simulink model "notch_tb_varTs"  (R2021a)
settings: Solver=VariableStepAuto  StartTime=0.0  StopTime=0.01  RelTol=1e-3
values from neighbouring files (symbols this model uses):
  FPGA_CLK_MHZ = 125    [lowpass_modelcomp_v1_0_setup.m]    (also in notch_modelcomp_v1_0_setup.m)
  maxSampleRate = 1e6    (= 1000000)    [lowpass_modelcomp_v1_0_setup.m]    (also in notch_modelcomp_v1_0_setup.m)
  notch_A0 = al0/be0    (= 0.984901734501)    [notch_modelcomp_v1_0_setup.m]
  notch_A1 = al1/be0    (= -1.87493826905)    [notch_modelcomp_v1_0_setup.m]
  notch_A2 = al2/be0    (= 0.984901734501)    [notch_modelcomp_v1_0_setup.m]
  notch_B1 = be1/be0    (= -1.87493826905)    [notch_modelcomp_v1_0_setup.m]
  notch_B2 = be2/be0    (= 0.969803469002)    [notch_modelcomp_v1_0_setup.m]
  samplePeriod = 1./SampleRate    (= 1e-05)    [lowpass_modelcomp_v1_0_setup.m]    (also in notch_modelcomp_v1_0_setup.m)
undefined symbols (not defined in the file or in its folder): xc7z030sbg485
libraries: hdlBasic x36, simulink x1, vmcUtilities x1, hdlUtilities x1
settings Model: Creator=osboxes  LastModifiedBy=valbas
settings SolverCC: AlgebraicLoopSolver=TrustRegion
settings DebuggingCC: SFMachineParentedDataDiag=warning

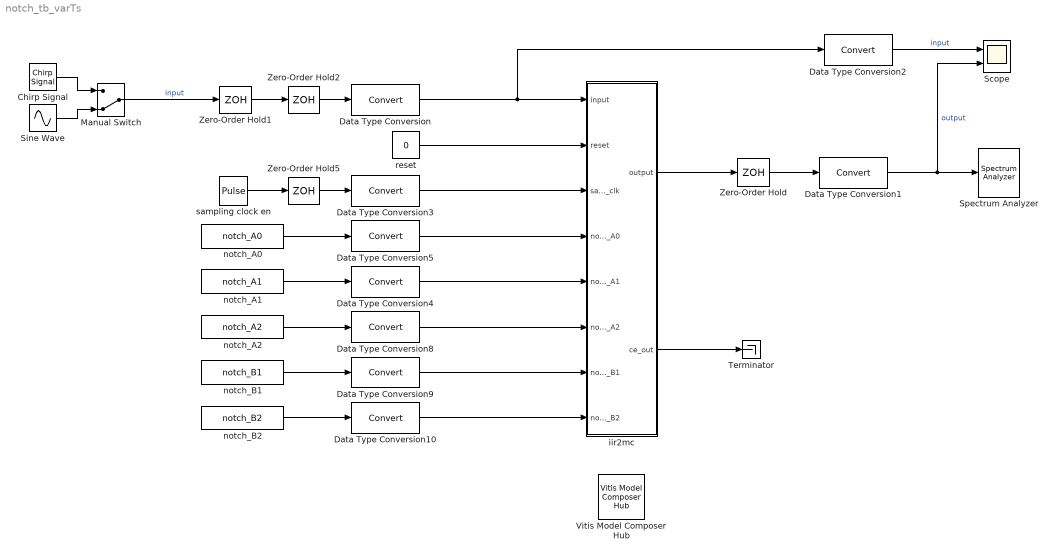
== system notch_tb_varTs ==
  Chirp Signal : simulink/Sources/Chirp Signal  f1=1  T=5  f2=1000
  Data Type Conversion{,1..2,4..5,8..10} (8 alike) : DataTypeConversion  RndMeth=Round
  Data Type Conversion3 : DataTypeConversion
  Manual Switch : ManualSwitch  CurrentSetting=0
  Scope : Scope  NumInputPorts=2
  Sine Wave : Sin  Amplitude=0.5  Frequency=4950*2*pi  SampleTime=0
  Spectrum Analyzer : SpectrumAnalyzer
  Terminator : Terminator
  Vitis Model Composer Hub : vmcUtilities/Vitis Model Composer Hub  Tag=genX  CodeGeneration=off  SubsystemName=iir2mc  TargetDirectory=./code  ExportType=HDL  IpVendor=xilinx.com  IpLibrary=hls  IpVersion=1.0  IpHWLanguage=Verilog  AieCompilerOptions={}  AieSimulatorOptions={}  CreateTestbench=off  TestbenchStackSize=10  RunRtlSim=off  RunCSim=off  RunAieSim=off  AieSimTimeout=50000  RunAieSimProfiling=off  LaunchVitisAnalyzer=off  PlotOutput=off  RunX86Sim=off  X86SimTimeout=10  GenHwImage=off  GenLibadfXo=off  PlatformType=Not Specified  HwSystemType=Baremetal  HwValidationTarget=hw  ProjDevice=xc7z030sbg485-1  ProjDevicePart=xc7z030sbg485-1  SamplePeriod=-1  ClockFrequency=200  DataPathParallelism=1  xilinxfamily=zynq  part=xc7z030  speed=-1  package=sbg485  directory=./netlist/ip/iir2mc/src  testbench=off  incr_netlist=off  synthesis_tool=Vivado  clock_wrapper=Clock Enables  dbl_ovrd=According to Block Masks  dcm_input_clock_period=10  sysclk_period=1.e3/FPGA_CLK_MHZ  simulink_period=1/(FPGA_CLK_MHZ*1.e6)  eval_field=0  IPInfoJsonString="{\"HDLSubsystem\":{\"SubsystemName\":\"iir2mc\",\"IPName\":\"iir2mc\",\"IPLibrary\":\"Panda_ModelComp\",\"IPVendor\":\"MaxIV\",\"IPVersion\":\"1.0\",\"TargetDirectory\":\"./netlist\",\"SubsystemDir\":\"./netlist/ip/iir2mc\"}}"  LogFileName=''  NThreads=4
  Zero-Order Hold : ZeroOrderHold  SampleTime=1/(FPGA_CLK_MHZ*1.e6)
  Zero-Order Hold1 : ZeroOrderHold  SampleTime=samplePeriod
  Zero-Order Hold2 : ZeroOrderHold  SampleTime=1/(FPGA_CLK_MHZ*1.e6)
  Zero-Order Hold5 : ZeroOrderHold  SampleTime=1/(FPGA_CLK_MHZ*1.e6)
  iir2mc : Subsystem
  notch_A0 : Constant  Value=notch_A0  OutDataTypeStr=double  SampleTime=1/(FPGA_CLK_MHZ*1.e6)
  notch_A1 : Constant  Value=notch_A1  OutDataTypeStr=double  SampleTime=1/(FPGA_CLK_MHZ*1.e6)
  notch_A2 : Constant  Value=notch_A2  OutDataTypeStr=double  SampleTime=1/(FPGA_CLK_MHZ*1.e6)
  notch_B1 : Constant  Value=notch_B1  OutDataTypeStr=double  SampleTime=1/(FPGA_CLK_MHZ*1.e6)
  notch_B2 : Constant  Value=notch_B2  OutDataTypeStr=double  SampleTime=1/(FPGA_CLK_MHZ*1.e6)
  reset : Constant  Value=0  OutDataTypeStr=boolean  SampleTime=1/(FPGA_CLK_MHZ*1.e6)
  sampling clock en : DiscretePulseGenerator  PulseType=Time based  Period=samplePeriod  PulseWidth=100/(samplePeriod*maxSampleRate)
  wires:
  Zero-Order Hold/1 -> Data Type Conversion1/1
  Zero-Order Hold2/1 -> Data Type Conversion/1
  reset/1 -> iir2mc/2(reset)
  iir2mc/1(output) -> Zero-Order Hold/1
  iir2mc/2(ce_out) -> Terminator/1
  Zero-Order Hold5/1 -> Data Type Conversion3/1
  Data Type Conversion3/1 -> iir2mc/3(sample_clk)
  notch_A0/1 -> Data Type Conversion5/1
  Data Type Conversion5/1 -> iir2mc/4(notch_A0)
  notch_A1/1 -> Data Type Conversion4/1
  Data Type Conversion4/1 -> iir2mc/5(notch_A1)
  notch_A2/1 -> Data Type Conversion8/1
  Data Type Conversion8/1 -> iir2mc/6(notch_A2)
  notch_B1/1 -> Data Type Conversion9/1
  Data Type Conversion9/1 -> iir2mc/7(notch_B1)
  notch_B2/1 -> Data Type Conversion10/1
  Data Type Conversion10/1 -> iir2mc/8(notch_B2)
  sampling clock en/1 -> Zero-Order Hold5/1
  Data Type Conversion/1 -> Data Type Conversion2/1, iir2mc/1(input)
  Data Type Conversion1/1 -> Scope/2, Spectrum Analyzer/1  "output"
  Sine Wave/1 -> Manual Switch/2
  Chirp Signal/1 -> Manual Switch/1
  Data Type Conversion2/1 -> Scope/1  "input"
  Zero-Order Hold1/1 -> Zero-Order Hold2/1
  Manual Switch/1 -> Zero-Order Hold1/1  "input"

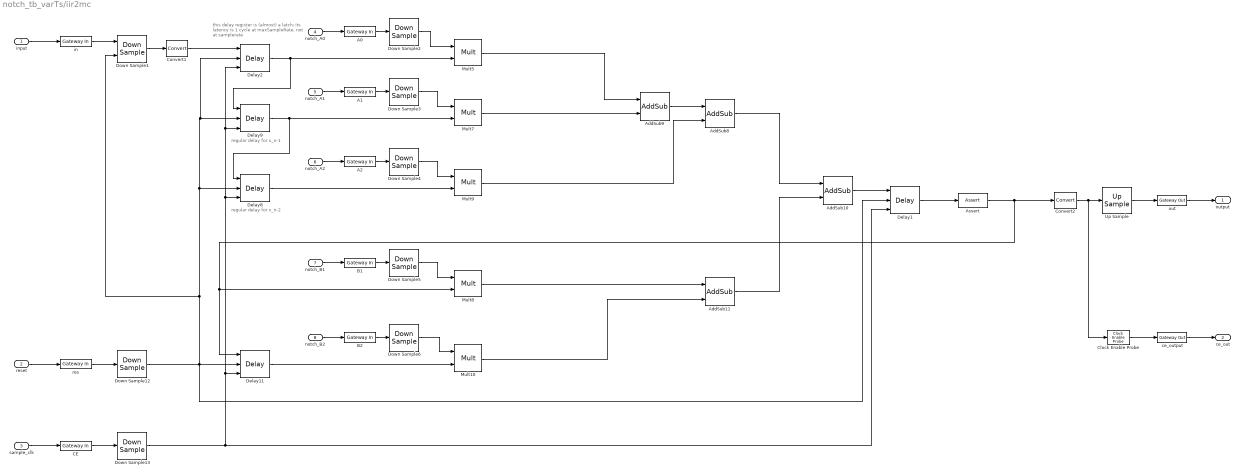
== system notch_tb_varTs/iir2mc ==
  note: regular delay for x_n-1
  note: this delay register is (almost) a latch;
      | its latency is 1 cycle at maxSampleRate,
      | not at samplerate
  note: regular delay for x_n-2
  input : Inport  OutDataTypeStr=fixdt(1,32,31)
  reset : Inport  Port=2
  sample_clk : Inport  Port=3  OutDataTypeStr=boolean
  notch_A0 : Inport  Port=4  OutDataTypeStr=single
  notch_A1 : Inport  Port=5  OutDataTypeStr=single
  notch_A2 : Inport  Port=6  OutDataTypeStr=single
  notch_B1 : Inport  Port=7  OutDataTypeStr=single
  notch_B2 : Inport  Port=8  OutDataTypeStr=single
  A0 : hdlBasic/Gateway In  gui_display_data_type=Floating-point  arith_type=Floating-point  n_bits=32  bin_pt=16  preci_type=Single  exp_width=8  frac_width=24  rows=1  columns=1  quantization="Round  (unbiased: +/- Inf)"  overflow=Saturate  period=1/(FPGA_CLK_MHZ*1.e6)  UseAsADC=off  ADCChannel='1'  interface=None  automatic_assignment=on  address_offset=hex2dec('00')  intf_name=''  intf_description=''  default_value=0  timing_constraint=None  locs_specified=off  LOCs={}  io_standard={}  inherit_from_input=off  hdl_port=on  XmcBlockStatus=1  maskContainerNames=group4  block_type=gatewayin  block_config=sysgen:gateway_in_config  block_width_w=590  block_height_w=620  block_width=640  block_height=850
  A1 : hdlBasic/Gateway In  gui_display_data_type=Floating-point  arith_type=Floating-point  n_bits=32  bin_pt=16  preci_type=Single  exp_width=8  frac_width=24  rows=1  columns=1  quantization="Round  (unbiased: +/- Inf)"  overflow=Saturate  period=1/(FPGA_CLK_MHZ*1.e6)  UseAsADC=off  ADCChannel='1'  interface=None  automatic_assignment=on  address_offset=hex2dec('00')  intf_name=''  intf_description=''  default_value=0  timing_constraint=None  locs_specified=off  LOCs={}  io_standard={}  inherit_from_input=off  hdl_port=on  XmcBlockStatus=1  maskContainerNames=group4  block_type=gatewayin  block_config=sysgen:gateway_in_config  block_width_w=590  block_height_w=620  block_width=640  block_height=850
  A2 : hdlBasic/Gateway In  gui_display_data_type=Floating-point  arith_type=Floating-point  n_bits=32  bin_pt=16  preci_type=Single  exp_width=8  frac_width=24  rows=1  columns=1  quantization="Round  (unbiased: +/- Inf)"  overflow=Saturate  period=1/(FPGA_CLK_MHZ*1.e6)  UseAsADC=off  ADCChannel='1'  interface=None  automatic_assignment=on  address_offset=hex2dec('00')  intf_name=''  intf_description=''  default_value=0  timing_constraint=None  locs_specified=off  LOCs={}  io_standard={}  inherit_from_input=off  hdl_port=on  XmcBlockStatus=1  maskContainerNames=group4  block_type=gatewayin  block_config=sysgen:gateway_in_config  block_width_w=590  block_height_w=620  block_width=640  block_height=850
  AddSub10 : hdlBasic/AddSub  mode=Subtraction  use_carryin=off  use_carryout=off  en=off  latency=0  precision=Full  arith_type="Signed  (2's comp)"  n_bits=62  bin_pt=40  quantization="Round  (unbiased: +/- Inf)"  overflow=Saturate  use_behavioral_HDL=off  hw_selection=Fabric  pipelined=off  XmcBlockStatus=1  maskContainerNames=tabcontainer1  block_type=addsub  block_config=sysgen:Addsub_config
  AddSub11 : hdlBasic/AddSub  mode=Addition  use_carryin=off  use_carryout=off  en=off  latency=0  precision=Full  arith_type="Signed  (2's comp)"  n_bits=62  bin_pt=40  quantization="Round  (unbiased: +/- Inf)"  overflow=Saturate  use_behavioral_HDL=off  hw_selection=Fabric  pipelined=off  XmcBlockStatus=1  maskContainerNames=tabcontainer1  block_type=addsub  block_config=sysgen:Addsub_config
  AddSub8 : hdlBasic/AddSub  mode=Addition  use_carryin=off  use_carryout=off  en=off  latency=0  precision=Full  arith_type=Unsigned  n_bits=16  bin_pt=14  quantization=Truncate  overflow=Wrap  use_behavioral_HDL=off  hw_selection=Fabric  pipelined=off  XmcBlockStatus=1  maskContainerNames=tabcontainer1  block_type=addsub  block_config=sysgen:Addsub_config
  AddSub9 : hdlBasic/AddSub  mode=Addition  use_carryin=off  use_carryout=off  en=off  latency=0  precision=Full  arith_type=Unsigned  n_bits=16  bin_pt=14  quantization=Truncate  overflow=Wrap  use_behavioral_HDL=off  hw_selection=Fabric  pipelined=off  XmcBlockStatus=1  maskContainerNames=tabcontainer1  block_type=addsub  block_config=sysgen:Addsub_config
  Assert : hdlBasic/Assert  assert_type=off  type_source=Explicitly  gui_display_data_type=Fixed-point  arith_type=Signed (2's comp)  n_bits=16  bin_pt=14  preci_type=Single  exp_width=8  frac_width=24  assert_rate=on  rate_source=Explicitly  period=1/maxSampleRate  output_port=on  XmcBlockStatus=1  maskContainerNames=group1  block_type=assert  block_config=sysgen:assert_config  block_width=609  block_height=900
  B1 : hdlBasic/Gateway In  gui_display_data_type=Floating-point  arith_type=Floating-point  n_bits=32  bin_pt=16  preci_type=Single  exp_width=8  frac_width=24  rows=1  columns=1  quantization="Round  (unbiased: +/- Inf)"  overflow=Saturate  period=1/(FPGA_CLK_MHZ*1.e6)  UseAsADC=off  ADCChannel='1'  interface=None  automatic_assignment=on  address_offset=hex2dec('00')  intf_name=''  intf_description=''  default_value=0  timing_constraint=None  locs_specified=off  LOCs={}  io_standard={}  inherit_from_input=off  hdl_port=on  XmcBlockStatus=1  maskContainerNames=group4  block_type=gatewayin  block_config=sysgen:gateway_in_config  block_width_w=590  block_height_w=620  block_width=640  block_height=850
  B2 : hdlBasic/Gateway In  gui_display_data_type=Floating-point  arith_type=Floating-point  n_bits=32  bin_pt=16  preci_type=Single  exp_width=8  frac_width=24  rows=1  columns=1  quantization="Round  (unbiased: +/- Inf)"  overflow=Saturate  period=1/(FPGA_CLK_MHZ*1.e6)  UseAsADC=off  ADCChannel='1'  interface=None  automatic_assignment=on  address_offset=hex2dec('00')  intf_name=''  intf_description=''  default_value=0  timing_constraint=None  locs_specified=off  LOCs={}  io_standard={}  inherit_from_input=off  hdl_port=on  XmcBlockStatus=1  maskContainerNames=group4  block_type=gatewayin  block_config=sysgen:gateway_in_config  block_width_w=590  block_height_w=620  block_width=640  block_height=850
  CE : hdlBasic/Gateway In  gui_display_data_type=Boolean  arith_type=Boolean  n_bits=16  bin_pt=14  preci_type=Single  exp_width=8  frac_width=24  rows=1  columns=1  quantization="Round  (unbiased: +/- Inf)"  overflow=Saturate  period=1/(FPGA_CLK_MHZ*1.e6)  UseAsADC=off  ADCChannel='1'  interface=None  automatic_assignment=on  address_offset=hex2dec('00')  intf_name=''  intf_description=''  default_value=0  timing_constraint=None  locs_specified=off  LOCs={}  io_standard={}  inherit_from_input=off  hdl_port=on  XmcBlockStatus=1  maskContainerNames=group4  block_type=gatewayin  block_config=sysgen:gateway_in_config  block_width_w=590  block_height_w=620  block_width=640  block_height=850
  Clock Enable Probe : hdlUtilities/Clock Enable Probe  inherit_constraints=on  XmcBlockStatus=1  maskContainerNames=group1  block_type=ceprobe  block_config=sysgen:CEProbe_config
  Convert1 : hdlBasic/Convert  gui_display_data_type=Floating-point  arith_type=Floating-point  n_bits=32  bin_pt=31  float_type=Single  exp_bits=8  fraction_bits=24  quantization=Truncate  overflow=Saturate  en=off  latency=0  pipeline=off  XmcBlockStatus=1  maskContainerNames=group2  block_type=convert  block_config=sysgen:Convert_config  block_width=595  block_height=885
  Convert2 : hdlBasic/Convert  gui_display_data_type=Fixed-point  arith_type=Signed (2's comp)  n_bits=32  bin_pt=31  float_type=Single  exp_bits=8  fraction_bits=24  quantization="Round  (unbiased: +/- Inf)"  overflow=Saturate  en=off  latency=0  pipeline=off  XmcBlockStatus=1  maskContainerNames=group2  block_type=convert  block_config=sysgen:Convert_config  block_width=595  block_height=885
  Delay{1..2,8..9,11} (5 alike) : hdlBasic/Delay  rst=on  en=on  latency=1  reg_retiming=off  XmcBlockStatus=1  maskContainerNames=group1  block_type=delay  block_config=sysgen:Delay_config
  Down Sample1 : hdlBasic/Down Sample  sample_ratio=FPGA_CLK_MHZ*1.e6/maxSampleRate  sample_phase="Last Value of Frame  (most efficient)"  en=off  rst=on  latency=1  XmcBlockStatus=1  maskContainerNames=group1  block_type=dsamp  block_config=sysgen:Downsample_config
  Down Sample{2..6,12..13} (7 alike) : hdlBasic/Down Sample  sample_ratio=FPGA_CLK_MHZ*1.e6/maxSampleRate  sample_phase="Last Value of Frame  (most efficient)"  en=off  rst=off  latency=1  XmcBlockStatus=1  maskContainerNames=group1  block_type=dsamp  block_config=sysgen:Downsample_config
  Mult10 : hdlBasic/Mult  precision=Full  arith_type="Signed  (2's comp)"  n_bits=41  bin_pt=21  quantization="Round  (unbiased: +/- Inf)"  overflow=Saturate  en=off  latency=0  use_behavioral_HDL=off  opt=Area  use_embedded=on  optimum_pipeline=off  pipeline=on  use_rpm=on  placement_style=Triangular  XmcBlockStatus=1  maskContainerNames=group1  block_type=mult  block_config=sysgen:Mult_config  block_width=598  block_height=876
  Mult5 : hdlBasic/Mult  precision=Full  arith_type="Signed  (2's comp)"  n_bits=16  bin_pt=14  quantization=Truncate  overflow=Wrap  en=off  latency=0  use_behavioral_HDL=off  opt=Area  use_embedded=on  optimum_pipeline=off  pipeline=on  use_rpm=on  placement_style=Triangular  XmcBlockStatus=1  maskContainerNames=group1  block_type=mult  block_config=sysgen:Mult_config  block_width=598  block_height=876
  Mult7 : hdlBasic/Mult  precision=Full  arith_type="Signed  (2's comp)"  n_bits=16  bin_pt=14  quantization=Truncate  overflow=Wrap  en=off  latency=0  use_behavioral_HDL=off  opt=Area  use_embedded=on  optimum_pipeline=off  pipeline=on  use_rpm=on  placement_style=Triangular  XmcBlockStatus=1  maskContainerNames=group1  block_type=mult  block_config=sysgen:Mult_config  block_width=598  block_height=876
  Mult8 : hdlBasic/Mult  precision=Full  arith_type="Signed  (2's comp)"  n_bits=41  bin_pt=21  quantization="Round  (unbiased: +/- Inf)"  overflow=Saturate  en=off  latency=0  use_behavioral_HDL=off  opt=Area  use_embedded=on  optimum_pipeline=off  pipeline=on  use_rpm=on  placement_style=Triangular  XmcBlockStatus=1  maskContainerNames=group1  block_type=mult  block_config=sysgen:Mult_config  block_width=598  block_height=876
  Mult9 : hdlBasic/Mult  precision=Full  arith_type="Signed  (2's comp)"  n_bits=16  bin_pt=14  quantization=Truncate  overflow=Wrap  en=off  latency=0  use_behavioral_HDL=off  opt=Area  use_embedded=on  optimum_pipeline=off  pipeline=on  use_rpm=on  placement_style=Triangular  XmcBlockStatus=1  maskContainerNames=group1  block_type=mult  block_config=sysgen:Mult_config  block_width=598  block_height=876
  Up Sample : hdlBasic/Up Sample  sample_ratio=FPGA_CLK_MHZ*1.e6/maxSampleRate  copy_samples=on  en=off  latency=1  XmcBlockStatus=1  maskContainerNames=group1  block_type=usamp  block_config=sysgen:Upsample_config
  ce_output : hdlBasic/Gateway Out  inherit_from_input=on  hdl_port=on  rows=1  columns=1  UseAsDAC=off  DACChannel='1'  interface=None  automatic_assignment=on  address_offset=hex2dec('00')  intf_name=''  intf_description=''  timing_constraint=Data Rate  locs_specified=off  LOCs={}  io_standard={}  XmcBlockStatus=1  maskContainerNames=group4  block_type=gatewayout  block_config=sysgen:gateway_out_config  block_width_w=590  block_height_w=620  block_width=620  block_height=750
  in : hdlBasic/Gateway In  gui_display_data_type=Fixed-point  arith_type=Signed (2's comp)  n_bits=32  bin_pt=31  preci_type=Single  exp_width=8  frac_width=24  rows=1  columns=1  quantization="Round  (unbiased: +/- Inf)"  overflow=Saturate  period=1/(FPGA_CLK_MHZ*1.e6)  UseAsADC=off  ADCChannel='1'  interface=None  automatic_assignment=on  address_offset=hex2dec('00')  intf_name=''  intf_description=''  default_value=0  timing_constraint=None  locs_specified=off  LOCs={}  io_standard={}  inherit_from_input=off  hdl_port=on  XmcBlockStatus=1  maskContainerNames=group4  block_type=gatewayin  block_config=sysgen:gateway_in_config  block_width_w=590  block_height_w=620  block_width=640  block_height=850
  out : hdlBasic/Gateway Out  inherit_from_input=on  hdl_port=on  rows=1  columns=1  UseAsDAC=off  DACChannel='1'  interface=None  automatic_assignment=on  address_offset=hex2dec('00')  intf_name=''  intf_description=''  timing_constraint=Data Rate  locs_specified=off  LOCs={}  io_standard={}  XmcBlockStatus=1  maskContainerNames=group4  block_type=gatewayout  block_config=sysgen:gateway_out_config  block_width_w=590  block_height_w=620  block_width=620  block_height=750
  res : hdlBasic/Gateway In  gui_display_data_type=Boolean  arith_type=Boolean  n_bits=16  bin_pt=14  preci_type=Single  exp_width=8  frac_width=24  rows=1  columns=1  quantization="Round  (unbiased: +/- Inf)"  overflow=Saturate  period=1/(FPGA_CLK_MHZ*1.e6)  UseAsADC=off  ADCChannel='1'  interface=None  automatic_assignment=on  address_offset=hex2dec('00')  intf_name=''  intf_description=''  default_value=0  timing_constraint=None  locs_specified=off  LOCs={}  io_standard={}  inherit_from_input=off  hdl_port=on  XmcBlockStatus=1  maskContainerNames=group4  block_type=gatewayin  block_config=sysgen:gateway_in_config  block_width_w=590  block_height_w=620  block_width=640  block_height=850
  output : Outport
  ce_out : Outport  Port=2
  wires:
  in/1 -> Down Sample1/1
  Convert2/1 -> Clock Enable Probe/1, Up Sample/1
  out/1 -> output/1
  ce_output/1 -> ce_out/1
  Up Sample/1 -> out/1
  res/1 -> Down Sample12/1
  Clock Enable Probe/1 -> ce_output/1
  input/1 -> in/1
  reset/1 -> res/1
  sample_clk/1 -> CE/1
  CE/1 -> Down Sample13/1
  Delay11/1 -> Mult10/2
  Delay2/1 -> Delay9/1, Mult5/2
  Mult9/1 -> AddSub8/2
  Mult5/1 -> AddSub9/1
  AddSub9/1 -> AddSub8/1
  Assert/1 -> Convert2/1, Mult8/2, Delay11/1
  Mult8/1 -> AddSub11/1
  Down Sample12/1 -> Down Sample1/2, Delay2/2, Delay9/2, Delay8/2, Delay11/2, Delay1/2
  Mult7/1 -> AddSub9/2
  AddSub11/1 -> AddSub10/2
  Down Sample2/1 -> Mult5/1
  Delay9/1 -> Delay8/1, Mult7/2
  Mult10/1 -> AddSub11/2
  AddSub8/1 -> AddSub10/1
  Delay8/1 -> Mult9/2
  A0/1 -> Down Sample2/1
  notch_A0/1 -> A0/1
  notch_A1/1 -> A1/1
  A1/1 -> Down Sample3/1
  Down Sample3/1 -> Mult7/1
  notch_A2/1 -> A2/1
  A2/1 -> Down Sample4/1
  Down Sample4/1 -> Mult9/1
  notch_B1/1 -> B1/1
  B1/1 -> Down Sample5/1
  Down Sample5/1 -> Mult8/1
  notch_B2/1 -> B2/1
  B2/1 -> Down Sample6/1
  Down Sample6/1 -> Mult10/1
  AddSub10/1 -> Delay1/1
  Delay1/1 -> Assert/1
  Down Sample13/1 -> Delay11/3, Delay8/3, Delay2/3, Delay9/3, Delay1/3
  Down Sample1/1 -> Convert1/1
  Convert1/1 -> Delay2/1
